simulink model "Target_Control_System"  (R2021b)
settings: Solver=FixedStepDiscrete  StartTime=0.0  StopTime=5  RelTol=1e-3
PreLoadFcn:
  | RTWConfigurationCB('preloadfcn', bdroot);
PostLoadFcn:
  | load('configuration/data_struct.mat');
  | load('configuration/fluxMaps_propMotor.mat');
  | load('configuration/parameterInit_PROP.mat');
  | load('configuration/parameterInit_PUMP.mat');
  | load('configuration/parameterInit_PITCH.mat');
  | load('configuration/parameterInit_TILT.mat');
  | %load('configuration/base_workspace_signal_definition.mat');
  | %load('resolvedatastores_to_baseworkspace_for_faster_simulation.mat');
model workspace (MAT data in the model file):
  SIMULATION_OPTIONS : Simulink.Parameter (value not decoded)
  TARGET_CODE_GEN : Simulink.Parameter (value not decoded)
  TCS_SAMPLE_FREQ_HZ : Simulink.Parameter (value not decoded)
symbols that are objects in the model workspace (value not decoded): TARGET_CODE_GEN, TCS_SAMPLE_FREQ_HZ
undefined symbols (not defined in the file): A_DQ_REF_LPF_INIT__PITCH, A_DQ_REF_LPF_INIT__PROP, A_DQ_REF_LPF_INIT__PUMP, A_DQ_REF_LPF_INIT__TILT, A_OBSERVER_CONFIDENCE_INIT__PITCH, A_OBSERVER_CONFIDENCE_INIT__PROP, A_OBSERVER_CONFIDENCE_INIT__PUMP, A_OBSERVER_CONFIDENCE_INIT__TILT, ACTUATOR_MAX_ANGLE_TRIP__PITCH, ACTUATOR_MIN_ANGLE_TRIP__PITCH, ACTUATOR_POS_SENSOR_INV_DIRECTION__PITCH, ACTUATOR_POS_SENSOR_INV_DIRECTION__TILT, ACTUATOR_POS_SENSOR_OFFSET__PITCH, ACTUATOR_POS_SENSOR_OFFSET__TILT, ADC_scaler1_baseaddr_TILT, ADC_SCALER_FLOAT_TO_FIXPOINT_EXPANSION, ANGLE_ELEC_FROM_SENSOR_OFFSET_INIT__PITCH, ANGLE_ELEC_FROM_SENSOR_OFFSET_INIT__PROP, ANGLE_ELEC_FROM_SENSOR_OFFSET_INIT__PUMP, ANGLE_ELEC_FROM_SENSOR_OFFSET_INIT__TILT, AUTO_CLEAR_FAULTS_ENABLED__PITCH, AUTO_CLEAR_FAULTS_ENABLED__PROP, AUTO_CLEAR_FAULTS_ENABLED__PUMP, AUTO_CLEAR_FAULTS_ENABLED__TILT, AUTO_CLEAR_FAULTS_WAIT_TICKS__PITCH, AUTO_CLEAR_FAULTS_WAIT_TICKS__PROP, AUTO_CLEAR_FAULTS_WAIT_TICKS__PUMP, AUTO_CLEAR_FAULTS_WAIT_TICKS__TILT, AUTO_I_ZERO_IDLE_TICKS__PITCH, AUTO_I_ZERO_IDLE_TICKS__PROP, AUTO_I_ZERO_IDLE_TICKS__PUMP, AUTO_I_ZERO_IDLE_TICKS__TILT, AUTO_I_ZERO_OFFSET_IDC_THRESHOLD__PITCH, AUTO_I_ZERO_OFFSET_IDC_THRESHOLD__PROP, AUTO_I_ZERO_OFFSET_IDC_THRESHOLD__PUMP, AUTO_I_ZERO_OFFSET_IDC_THRESHOLD__TILT, AUTO_I_ZERO_OFFSET_IPH_THRESHOLD__PITCH, AUTO_I_ZERO_OFFSET_IPH_THRESHOLD__PROP, AUTO_I_ZERO_OFFSET_IPH_THRESHOLD__PUMP, AUTO_I_ZERO_OFFSET_IPH_THRESHOLD__TILT, AUTO_SENSORLESS_SWITCHOVER_DISABLE_OMEGA, AUTO_SENSORLESS_SWITCHOVER_ENABLE_OMEGA, AUTO_SENSORLESS_SWITCHOVER_MIN_CONFIDENCE, AUXILIARY_PROTECTION_UNIT_BASEADDR__TILT, blanking_max_error_omega_INIT_PITCH, blanking_max_error_omega_INIT_TILT, blanking_max_error_position_INIT_PITCH, blanking_max_error_position_INIT_TILT, BRUTE_START_I_Q_REF_RAMP_SPEED__PITCH, BRUTE_START_I_Q_REF_RAMP_SPEED__PROP, BRUTE_START_I_Q_REF_RAMP_SPEED__PUMP, BRUTE_START_I_Q_REF_RAMP_SPEED__TILT, CONTROL_LOOP_DT_INIT__PITCH, CONTROL_LOOP_DT_INIT__PROP, CONTROL_LOOP_DT_INIT__PUMP, CONTROL_LOOP_DT_INIT__TILT, CORRECTION_FILTER_SCALE__PITCH, CORRECTION_FILTER_SCALE__PROP, CORRECTION_FILTER_SCALE__PUMP, CORRECTION_FILTER_SCALE__TILT ... (+458)
libraries: simulink x178, Reusables_Lib x24
(part 38 of 47)

== system Target_Control_System/Target_Control_System/MainLoop/tiltMotor_mainLoop/Decimation gate for 200 Hz Tilt/motorTaskMainDecimationAStep(&oTilt)/Forced current injection for broken input sensors/Enabled Subsystem/Rudimentary_forced_angle_position_control ==
  note: // (fErrorReduction_ assumed to be gte 0)
  note: // Limit maximum speed
  note: // Reduce top speed 33-fold
  Enable : EnablePort
  Abs : Abs
  Add : Sum  Inputs=+-
  Add1 : Sum  Inputs=+-
  Data Store Read10 : DataStoreRead  DataStoreName=oTilt  DataStoreElements=oTilt.oMot_.oState_.oPosSensor_.oPidDataPosCtrl_.oParameter_.fOutMax_  IndexOptions=Index vector (dialog)  Indices=1  OutputSizes=1
  Data Store Read11 : DataStoreRead  DataStoreName=oTilt  DataStoreElements=oTilt.oMot_.oState_.oPosSensor_.oPidDataPosCtrl_.oParameter_.fOutMin_  IndexOptions=Index vector (dialog)  Indices=1  OutputSizes=1
  Data Store Read6 : DataStoreRead  DataStoreName=oTilt  DataStoreElements=oTilt.oMot_.oState_.oRampDataPos_.fRampOut_  IndexOptions=Index vector (dialog)  Indices=1  OutputSizes=1
  Data Store Read7 : DataStoreRead  DataStoreName=oTilt  DataStoreElements=oTilt.oMot_.oState_.oPosSensor_.fActuatorAngleFromSensor_  IndexOptions=Index vector (dialog)  Indices=1  OutputSizes=1
  Data Store Read8 : DataStoreRead  DataStoreName=oTilt  DataStoreElements=oTilt.oMot_.oState_.oPosSensor_.oPidDataPosCtrl_.oParameter_.fErrorReduction_  IndexOptions=Index vector (dialog)  Indices=1  OutputSizes=1
  Data Store Read9 : DataStoreRead  DataStoreName=oTilt  DataStoreElements=oTilt.oMot_.oState_.oPosSensor_.oPidDataPosCtrl_.oParameter_.fKp_  IndexOptions=Index vector (dialog)  Indices=1  OutputSizes=1
  Data Store Write4 : DataStoreWrite  DataStoreName=oTilt  DataStoreElements=oTilt.oMot_.oState_.oRampDataOmegaERef_.fSetpoint_  IndexOptions=Index vector (dialog)  Indices=1  OutputSizes=1
  Divide : Product  Inputs=**
  Divide1 : Product  Inputs=**
  Gain : Gain  Gain=0.03
  Gain1 : Gain  Gain=0.03
  Max : MinMax  Function=max  Inputs=2
  Min : MinMax  Inputs=2
  Saturation : Saturate  UpperLimit=inf  LowerLimit=0
  Sign : Signum
  wires:
  Data Store Read10/1 -> Gain/1
  Gain/1 -> Min/2
  Data Store Read9/1 -> Divide1/2
  Divide1/1 -> Min/1  "fOmegaRef"
  Sign/1 -> Divide/1
  Data Store Read11/1 -> Gain1/1
  Saturation/1 -> Divide/2
  Min/1 -> Max/1
  Gain1/1 -> Max/2
  Data Store Read7/1 -> Add/2
  Add1/1 -> Saturation/1  "fTemp"
  Data Store Read8/1 -> Add1/2
  Add/1 -> Abs/1, Sign/1  "fPositionError"
  Divide/1 -> Divide1/1  "fPositionError"
  Data Store Read6/1 -> Add/1
  Abs/1 -> Add1/1
  Max/1 -> Data Store Write4/1

== system Target_Control_System/Target_Control_System/MainLoop/tiltMotor_mainLoop/Decimation gate for 200 Hz Tilt/motorTaskMainDecimationAStep(&oTilt)/Idle controller/Not forced angle/piControllerStep_Idle_Controller(&oTilt) ==
  fActual : Inport
  fTarget : Inport  Port=2
  fKp : Inport  Port=3
  fKi : Inport  Port=4
  fScale : Inport  Port=5
  fLoopDt : Inport  Port=6
  fIntMax : Inport  Port=7
  fOutMax : Inport  Port=8
  fIntMin : Inport  Port=9
  fOutMin : Inport  Port=10
  fState : Inport  Port=11
  Add : Sum  Inputs=|++
  Mux : Mux  Inputs=3
  Mux1 : Mux  Inputs=3
  Product : Product
  Saturation Dynamic : simulink/Discontinuities/Saturation Dynamic  OutMin=[]  OutMax=[]  OutDataTypeStr=Inherit: Same as second input  OutDataType=fixdt(1, 16)  OutScaling=2^-10  DoSatur=off
  Saturation Dynamic1 : simulink/Discontinuities/Saturation Dynamic  OutMin=[]  OutMax=[]  OutDataTypeStr=Inherit: Same as second input  OutDataType=fixdt(1, 16)  OutScaling=2^-10  DoSatur=off
  Scope3 : Scope  NumInputPorts=6
  Sum1 : Sum  Inputs=++|
  Sum22 : Sum  Inputs=-+|
  Unit Delay2 : UnitDelay  SampleTime=-1  HasFrameUpgradeWarning=on
  fError * fKi_ * fScale : Fcn  Expr=u(1)*u(2)*u(3)
  fError * fKp_ * fScale1 : Fcn  Expr=u(1)*u(2)*u(3)
  fOutput : Outport
  *fpState : Outport  Port=2
  wires:
  fLoopDt/1 -> Product/2
  fOutMax/1 -> Saturation Dynamic1/1
  fOutMin/1 -> Saturation Dynamic1/3
  fIntMin/1 -> Saturation Dynamic/3
  fIntMax/1 -> Saturation Dynamic/1
  Unit Delay2/1 -> Scope3/5, *fpState/1, Sum1/2
  Add/1 -> Saturation Dynamic/2
  fState/1 -> Add/2
  Product/1 -> Add/1
  Mux1/1 -> fError * fKp_ * fScale1/1
  fKi/1 -> Mux/2
  fScale/1 -> Mux/1, Mux1/3
  fKp/1 -> Mux1/2
  Mux/1 -> fError * fKi_ * fScale/1
  Saturation Dynamic1/1 -> fOutput/1, Scope3/6
  Sum1/1 -> Saturation Dynamic1/2  "fError"
  fError * fKp_ * fScale1/1 -> Sum1/1, Scope3/4
  Saturation Dynamic/1 -> Unit Delay2/1  "*fpState"
  fActual/1 -> Sum22/1, Scope3/2
  fTarget/1 -> Sum22/2, Scope3/1
  fError * fKi_ * fScale/1 -> Product/1
  Sum22/1 -> Scope3/3, Mux/3, Mux1/1  "fError"

== system Target_Control_System/Target_Control_System/MainLoop/tiltMotor_mainLoop/Decimation gate for 200 Hz Tilt/motorTaskMainDecimationAStep(&oTilt)/Position control checks/Position control mode/Check AD2S1210 ==
  function : TriggerPort  TriggerType=function-call  VariantControl=Variant
  Data Store Read : DataStoreRead  DataStoreName=oTilt  DataStoreElements=oTilt.oMot_.oState_.oPosSensor_.eInputPositionSensorType_  IndexOptions=Index vector (dialog)  Indices=1  OutputSizes=1
  Enabled Subsystem : Subsystem  TreatAsAtomicUnit=on
  Enumerated Constant : simulink/Sources/Enumerated Constant  OutDataTypeStr=Enum: EPositionSensor_t  Value=EPositionSensor_t.eResolver  SampleTime=-1
  Equal : RelationalOperator  Operator===  OutDataTypeStr=boolean  RndMeth=Simplest
  wires:
  Equal/1 -> Enabled Subsystem/Enable
  Data Store Read/1 -> Equal/1
  Enumerated Constant/1 -> Equal/2

== system Target_Control_System/Target_Control_System/MainLoop/tiltMotor_mainLoop/Decimation gate for 200 Hz Tilt/motorTaskMainDecimationAStep(&oTilt)/Position control checks/Position control mode/Check fighting controllers ==
  note: Check fighting controllers
      | (For dual inverter independent position control)
      | MvdG: Possibly remove again, because it is not actually in use? QAZ
  note: (ab)use the threshold setting as on-off switch too.
  function : TriggerPort  TriggerType=function-call  VariantControl=Variant
  Constant : Constant  Value=0  OutDataTypeStr=int32  SampleTime=-1
  Data Store Read : DataStoreRead  DataStoreName=oTilt  DataStoreElements=oTilt.oMot_.oState_.oPosSensor_.fFightingCurrentMagnitude_  IndexOptions=Index vector (dialog)  Indices=1  OutputSizes=1
  Enabled Subsystem : Subsystem  TreatAsAtomicUnit=on
  GreaterThan : RelationalOperator  Operator=>  OutDataTypeStr=boolean  RndMeth=Simplest
  wires:
  Constant/1 -> GreaterThan/2
  GreaterThan/1 -> Enabled Subsystem/Enable
  Data Store Read/1 -> GreaterThan/1

== system Target_Control_System/Target_Control_System/MainLoop/tiltMotor_mainLoop/Decimation gate for 200 Hz Tilt/motorTaskMainDecimationAStep(&oTilt)/Position control checks/Position control mode/Check for position halted ==
  function : TriggerPort  TriggerType=function-call  VariantControl=Variant
  Chart1 : Stateflow chart  TreatAsAtomicUnit=on

== system Target_Control_System/Target_Control_System/MainLoop/tiltMotor_mainLoop/Decimation gate for 200 Hz Tilt/motorTaskMainDecimationAStep(&oTilt)/Position control checks/Position control mode/checkSensorLimits(&oTilt) ==
  note: In the emergency 'ePassiveHolding' mode, iPosControlEnabled_ is false, so this will not trip
  function : TriggerPort  TriggerType=function-call  VariantControl=Variant
  Check broken sensor : Subsystem  TreatAsAtomicUnit=on
  Check delta input-output : Subsystem  TreatAsAtomicUnit=on
  Check for stuck sensor : Subsystem  TreatAsAtomicUnit=on
  Check limits : Subsystem  TreatAsAtomicUnit=on
  Function-Call Generator : simulink/Ports & Subsystems/Function-Call Generator  sample_time=-1  numberOfIterations=1  DisallowWideOutput=off
  Function-Call Split{1..3,10} (4 alike) : FunctionCallSplit  NumOutputPorts=2
  Read sensor flags : Subsystem  TreatAsAtomicUnit=on
  wires:
  Function-Call Split2/2 -> Function-Call Split3/1
  Function-Call Split10/1 -> Read sensor flags/Trigger
  Function-Call Split1/1 -> Check limits/Trigger
  Function-Call Split3/2 -> Check for stuck sensor/Trigger
  Function-Call Split1/2 -> Function-Call Split2/1
  Function-Call Split2/1 -> Check broken sensor/Trigger
  Function-Call Generator/1 -> Function-Call Split10/1
  Function-Call Split3/1 -> Check delta input-output/Trigger
  Function-Call Split10/2 -> Function-Call Split1/1

== system Target_Control_System/Target_Control_System/MainLoop/tiltMotor_mainLoop/Decimation gate for 5000 Hz Tilt/motorTaskProcessExternalSetpoints(&oTilt)/set_target/Id_target/Subsystem ==
  Input : Inport
  Enable : EnablePort
  Data Store Read1 : DataStoreRead  DataStoreName=oTilt  DataStoreElements=oTilt.oMot_.oParam_.fISetpointMax_  IndexOptions=Index vector (dialog)  Indices=1  OutputSizes=1
  Data Store Read74 : DataStoreRead  DataStoreName=oTilt  DataStoreElements=oTilt.oMot_.oParam_.fISetpointMax_  IndexOptions=Index vector (dialog)  Indices=1  OutputSizes=1
  Data Store Write1 : DataStoreWrite  DataStoreName=oTilt  DataStoreElements=oTilt.oMot_.oState_.fIdExternalSetpoint_  IndexOptions=Index vector (dialog)  Indices=1  OutputSizes=1
  Gain2 : Gain  Gain=-1
  Saturation Dynamic : simulink/Discontinuities/Saturation Dynamic  OutMin=[]  OutMax=[]  OutDataTypeStr=Inherit: Same as second input  OutDataType=fixdt(1, 16)  OutScaling=2^-10  DoSatur=off
  wires:
  Data Store Read1/1 -> Gain2/1
  Data Store Read74/1 -> Saturation Dynamic/1
  Gain2/1 -> Saturation Dynamic/3
  Input/1 -> Saturation Dynamic/2
  Saturation Dynamic/1 -> Data Store Write1/1

== system Target_Control_System/Target_Control_System/MainLoop/tiltMotor_mainLoop/Decimation gate for 5000 Hz Tilt/motorTaskProcessExternalSetpoints(&oTilt)/set_target/Iq_target/Subsystem ==
  Enable : EnablePort
  Data Store Read1 : DataStoreRead  DataStoreName=oTilt  DataStoreElements=oTilt.oMot_.oParam_.fIqSetpointMax_  IndexOptions=Index vector (dialog)  Indices=1  OutputSizes=1
  Data Store Read68 : DataStoreRead  DataStoreName=oTilt  DataStoreElements=oTilt.oMot_.oIn_.fIqSetpoint_  IndexOptions=Index vector (dialog)  Indices=1  OutputSizes=1
  Data Store Read74 : DataStoreRead  DataStoreName=oTilt  DataStoreElements=oTilt.oMot_.oParam_.fIqSetpointMax_  IndexOptions=Index vector (dialog)  Indices=1  OutputSizes=1
  Data Store Read81 : DataStoreRead  DataStoreName=oTilt  DataStoreElements=oTilt.oMot_.oParam_.fDynILimIntegratorLeakageFactor_  IndexOptions=Index vector (dialog)  Indices=1  OutputSizes=1
  Data Store Write19 : DataStoreWrite  DataStoreName=oTilt  DataStoreElements=oTilt.oMot_.oState_.fIqRefBeforeRamp_  IndexOptions=Index vector (dialog)  Indices=1  OutputSizes=1
  Dynamic Current Limiting Tilt : Subsystem  TreatAsAtomicUnit=on
  Gain2 : Gain  Gain=-1
  Saturation Dynamic : simulink/Discontinuities/Saturation Dynamic  OutMin=[]  OutMax=[]  OutDataTypeStr=Inherit: Same as second input  OutDataType=fixdt(1, 16)  OutScaling=2^-10  DoSatur=off
  Switch4 : Switch  Criteria=u2 > Threshold
  wires:
  Dynamic Current Limiting Tilt/1(fIqRefBeforeRamp_) -> Switch4/1
  Switch4/1 -> Data Store Write19/1
  Data Store Read81/1 -> Dynamic Current Limiting Tilt/Enable, Switch4/2
  Gain2/1 -> Saturation Dynamic/3
  Data Store Read74/1 -> Saturation Dynamic/1
  Data Store Read68/1 -> Saturation Dynamic/2
  Data Store Read1/1 -> Gain2/1
  Saturation Dynamic/1 -> Switch4/3

== system Target_Control_System/Target_Control_System/MainLoop/tiltMotor_mainLoop/Decimation gate for 5000 Hz Tilt/motorTaskProcessExternalSetpoints(&oTilt)/set_target/position_target/Subsystem ==
  Enable : EnablePort
  Data Store Read2 : DataStoreRead  DataStoreName=oTilt  DataStoreElements=oTilt.oMot_.oIn_.fPosSetpoint_  IndexOptions=Index vector (dialog)  Indices=1  OutputSizes=1
  Data Store Read85 : DataStoreRead  DataStoreName=oTilt  DataStoreElements=oTilt.oMot_.oState_.uiDriveState_  IndexOptions=Index vector (dialog)  Indices=1  OutputSizes=1
  Data Store Write1 : DataStoreWrite  DataStoreName=oTilt  DataStoreElements=oTilt.oMot_.oState_.oRampDataPos_.fSetpoint_  IndexOptions=Index vector (dialog)  Indices=1  OutputSizes=1
  Equal13 : RelationalOperator  Operator=~=  OutDataTypeStr=boolean  RndMeth=Simplest
  Position Limiting Tilt : Subsystem  TreatAsAtomicUnit=on
  const17 : Constant  Value=228  OutDataTypeStr=uint32  SampleTime=-1
  wires:
  Equal13/1 -> Position Limiting Tilt/Enable
  const17/1 -> Equal13/1
  Data Store Read85/1 -> Equal13/2
  Data Store Read2/1 -> Data Store Write1/1, Position Limiting Tilt/1(oRampDataPos_.fSetpoint_)

== system Target_Control_System/Target_Control_System/MainLoop/tiltMotor_mainLoop/Decimation gate for 5000 Hz Tilt/motorTaskProcessExternalSetpoints(&oTilt)/set_target/speed_target/Subsystem ==
  Enable : EnablePort
  Data Store Read1 : DataStoreRead  DataStoreName=oTilt  DataStoreElements=oTilt.oMot_.oParam_.fPolePairs_  IndexOptions=Index vector (dialog)  Indices=1  OutputSizes=1
  Data Store Read2 : DataStoreRead  DataStoreName=oTilt  DataStoreElements=oTilt.oMot_.oIn_.fRpmSetpoint_  IndexOptions=Index vector (dialog)  Indices=1  OutputSizes=1
  Data Store Read3 : DataStoreRead  DataStoreName=oTilt  DataStoreElements=oTilt.oMot_.oParam_.fOmegaESetpointMax_  IndexOptions=Index vector (dialog)  Indices=1  OutputSizes=1
  Data Store Read74 : DataStoreRead  DataStoreName=oTilt  DataStoreElements=oTilt.oMot_.oParam_.fOmegaESetpointMax_  IndexOptions=Index vector (dialog)  Indices=1  OutputSizes=1
  Data Store Write1 : DataStoreWrite  DataStoreName=oTilt  DataStoreElements=oTilt.oMot_.oState_.oRampDataOmegaERef_.fSetpoint_  IndexOptions=Index vector (dialog)  Indices=1  OutputSizes=1
  Gain : Gain  Gain=-1
  Product : Product  Inputs=3
  Saturation Dynamic : simulink/Discontinuities/Saturation Dynamic  OutMin=[]  OutMax=[]  OutDataTypeStr=Inherit: Same as second input  OutDataType=fixdt(1, 16)  OutScaling=2^-10  DoSatur=off
  const1 : Constant  Value=0.10471975512  OutDataTypeStr=single  SampleTime=-1
  wires:
  Saturation Dynamic/1 -> Data Store Write1/1
  Product/1 -> Saturation Dynamic/2
  Data Store Read3/1 -> Gain/1
  Gain/1 -> Saturation Dynamic/3
  Data Store Read74/1 -> Saturation Dynamic/1
  const1/1 -> Product/2
  Data Store Read1/1 -> Product/3
  Data Store Read2/1 -> Product/1

== system Target_Control_System/Target_Control_System/MainLoop/tiltMotor_mainLoop/mainTask_tilt/motorTaskMainFastStep(&oTilt)/Automatic switching to sensorless - Tilt/Automatic switching to sensorless/Switch to sensored  ==
  note: // Presently enabled, do we need to disable?
  fObserverConfidence : Inport
  Action Port : ActionPort
  Abs2 : Abs
  Data Store Read1 : DataStoreRead  DataStoreName=oTilt  DataStoreElements=oTilt.oMot_.oIn_.fOmegaEObserverRaw2_  IndexOptions=Index vector (dialog)  Indices=1  OutputSizes=1
  Data Store Read2 : DataStoreRead  DataStoreName=oTilt  DataStoreElements=oTilt.oMot_.oParam_.fAutoSensorlessSwitchoverDisableOmega_  IndexOptions=Index vector (dialog)  Indices=1  OutputSizes=1
  Data Store Read3 : DataStoreRead  DataStoreName=oTilt  DataStoreElements=oTilt.oMot_.oParam_.fAutoSensorlessSwitchoverMinConfidence_  IndexOptions=Index vector (dialog)  Indices=1  OutputSizes=1
  Less Than2 : RelationalOperator  Operator=<  OutDataTypeStr=boolean  RndMeth=Simplest
  Less Than3 : RelationalOperator  Operator=<  OutDataTypeStr=boolean  RndMeth=Simplest
  OR1 : Logic  Operator=OR  AllPortsSameDT=off  OutDataTypeStr=boolean
  Switch to sensored : Subsystem  TreatAsAtomicUnit=on
  wires:
  Data Store Read2/1 -> Less Than2/2
  Data Store Read3/1 -> Less Than3/2
  OR1/1 -> Switch to sensored/Enable
  Less Than3/1 -> OR1/2
  fObserverConfidence/1 -> Less Than3/1
  Abs2/1 -> Less Than2/1
  Less Than2/1 -> OR1/1
  Data Store Read1/1 -> Abs2/1

== system Target_Control_System/Target_Control_System/MainLoop/tiltMotor_mainLoop/mainTask_tilt/motorTaskMainFastStep(&oTilt)/Automatic switching to sensorless - Tilt/Automatic switching to sensorless/Switch to sensorless? ==
  fObserverConfidence : Inport
  Action Port : ActionPort
  Abs2 : Abs
  Data Store Read1 : DataStoreRead  DataStoreName=oTilt  DataStoreElements=oTilt.oMot_.oIn_.fOmegaEObserverRaw2_  IndexOptions=Index vector (dialog)  Indices=1  OutputSizes=1
  Data Store Read2 : DataStoreRead  DataStoreName=oTilt  DataStoreElements=oTilt.oMot_.oParam_.fAutoSensorlessSwitchoverEnableOmega_  IndexOptions=Index vector (dialog)  Indices=1  OutputSizes=1
  Data Store Read3 : DataStoreRead  DataStoreName=oTilt  DataStoreElements=oTilt.oMot_.oParam_.fAutoSensorlessSwitchoverMinConfidence_  IndexOptions=Index vector (dialog)  Indices=1  OutputSizes=1
  Less Than2 : RelationalOperator  Operator=>  OutDataTypeStr=boolean  RndMeth=Simplest
  Less Than3 : RelationalOperator  Operator=>  OutDataTypeStr=boolean  RndMeth=Simplest
  OR1 : Logic  AllPortsSameDT=off  OutDataTypeStr=boolean
  Switch to sensorless : Subsystem  TreatAsAtomicUnit=on
  wires:
  OR1/1 -> Switch to sensorless/Enable
  Data Store Read3/1 -> Less Than3/2
  Less Than2/1 -> OR1/1
  Data Store Read2/1 -> Less Than2/2
  Data Store Read1/1 -> Abs2/1
  Abs2/1 -> Less Than2/1
  fObserverConfidence/1 -> Less Than3/1
  Less Than3/1 -> OR1/2

== system Target_Control_System/Target_Control_System/MainLoop/tiltMotor_mainLoop/mainTask_tilt/motorTaskMainFastStep(&oTilt)/Control Loops - Tilt/Position Controller Tilt/Connect PosController to CurrentController ==
  fPMultiplier : Inport
  fIMultiplier : Inport  Port=2
  DMultiplier : Inport  Port=3
  fITerm : Inport  Port=4
  fDTerm : Inport  Port=5
  fPTerm : Inport  Port=6
  Add : Sum  Inputs=+++
  Divide : Product  Inputs=**
  Divide1 : Product  Inputs=**
  Divide2 : Product  Inputs=**
  fIqRefFromSpeedController : Outport
  wires:
  Add/1 -> fIqRefFromSpeedController/1
  Divide2/1 -> Add/3
  Divide/1 -> Add/1
  Divide1/1 -> Add/2
  fDTerm/1 -> Divide2/1
  DMultiplier/1 -> Divide2/2
  fITerm/1 -> Divide1/1
  fIMultiplier/1 -> Divide1/2
  fPMultiplier/1 -> Divide/2
  fPTerm/1 -> Divide/1

== system Target_Control_System/Target_Control_System/MainLoop/tiltMotor_mainLoop/mainTask_tilt/motorTaskMainFastStep(&oTilt)/Control Loops - Tilt/Position Controller Tilt/pid2ControllerStep(oPidDataPosCtrl)_pitch ==
  fTarget : Inport
  fActual : Inport  Port=2
  fErrorReduction : Inport  Port=3
  fLargeErrorThresholdPositive : Inport  Port=4
  fLargeErrorThresholdNegative : Inport  Port=5
  fBlankingMaxError : Inport  Port=6
  fKi : Inport  Port=7
  ipInhibitTarget : Inport  Port=8
  fLoopDt : Inport  Port=9
  fIntMax : Inport  Port=10
  fIntMin : Inport  Port=11
  fIntegratorLeakFactor : Inport  Port=12
  fKd : Inport  Port=13
  fActualDt : Inport  Port=14
  fDMax : Inport  Port=15
  fDMin : Inport  Port=16
  fKp : Inport  Port=17
  fOutMax : Inport  Port=18
  fOutMin : Inport  Port=19
  fpState : Inport  Port=20
  Abs : Abs
  Abs1 : Abs
  Add : Sum  Inputs=|++
  Add1 : Sum
  Constant : Constant  Value=0  OutDataTypeStr=single  SampleTime=-1
  Constant3 : Constant  Value=0  OutDataTypeStr=single  SampleTime=-1
  Constant4 : Constant  Value=0  OutDataTypeStr=single  SampleTime=-1
  Constant5 : Constant  OutDataTypeStr=single  SampleTime=-1
  Constant6 : Constant  OutDataTypeStr=int32  SampleTime=-1
  Constant7 : Constant  Value=-1  OutDataTypeStr=int32  SampleTime=-1
  Constant8 : Constant  Value=0  OutDataTypeStr=int32  SampleTime=-1
  Divide : Product  Inputs=**
  Divide1 : Product  Inputs=**
  GreaterThan2 : RelationalOperator  OutDataTypeStr=boolean  RndMeth=Simplest
  GreaterThan3 : RelationalOperator  Operator=>  OutDataTypeStr=boolean  RndMeth=Simplest
  GreaterThan4 : RelationalOperator  Operator=>  OutDataTypeStr=boolean  RndMeth=Simplest
  GreaterThan5 : RelationalOperator  Operator=<  OutDataTypeStr=boolean  RndMeth=Simplest
  GreaterThan6 : RelationalOperator  Operator=<  OutDataTypeStr=boolean  RndMeth=Simplest
  GreaterThan7 : RelationalOperator  Operator=>  OutDataTypeStr=boolean  RndMeth=Simplest
  GreaterThan8 : RelationalOperator  Operator=<  OutDataTypeStr=boolean  RndMeth=Simplest
  OR1 : Logic  AllPortsSameDT=off  OutDataTypeStr=boolean
  OR2 : Logic  AllPortsSameDT=off  OutDataTypeStr=boolean
  OR3 : Logic  Operator=OR  AllPortsSameDT=off  OutDataTypeStr=boolean
  Product{,1..4} (5 alike) : Product
  Saturation : Saturate  UpperLimit=inf  LowerLimit=0
  Saturation Dynamic : simulink/Discontinuities/Saturation Dynamic  OutMin=[]  OutMax=[]  OutDataTypeStr=Inherit: Same as second input  OutDataType=fixdt(1, 16)  OutScaling=2^-10  DoSatur=off
  Saturation Dynamic1 : simulink/Discontinuities/Saturation Dynamic  OutMin=[]  OutMax=[]  OutDataTypeStr=Inherit: Same as second input  OutDataType=fixdt(1, 16)  OutScaling=2^-10  DoSatur=off
  Saturation Dynamic2 : simulink/Discontinuities/Saturation Dynamic  OutMin=[]  OutMax=[]  OutDataTypeStr=Inherit: Same as second input  OutDataType=fixdt(1, 16)  OutScaling=2^-10  DoSatur=off
  Scope : Scope  NumInputPorts=4
  Sign : Signum
  Sum : Sum  Inputs=|++
  Sum2 : Sum  Inputs=-+|
  Sum22 : Sum  Inputs=-+|
  Sum4 : Sum  Inputs=+-|
  Switch{1..4} (4 alike) : Switch  Criteria=u2 > Threshold
  Unit Delay2 : UnitDelay  SampleTime=-1  HasFrameUpgradeWarning=on
  iLargeErrorPresent : Outport
  fITerm : Outport  Port=2
  fDTerm : Outport  Port=3
  fPTerm : Outport  Port=4
  fOutput : Outport  Port=5
  *fpState : Outport  Port=6
  wires:
  Switch3/1 -> iLargeErrorPresent/1
  Constant6/1 -> Switch4/1
  GreaterThan8/1 -> Switch3/2
  GreaterThan7/1 -> Switch4/2
  Switch4/1 -> Switch3/3
  Constant8/1 -> Switch4/3
  Constant7/1 -> Switch3/1
  Sum/1 -> Saturation Dynamic1/2, Scope/2
  Add1/1 -> Sum/2
  Product4/1 -> fPTerm/1, Sum/1
  fKp/1 -> Product4/1
  Saturation Dynamic2/1 -> fDTerm/1, Add1/1  "fDTerm"
  fDMax/1 -> Saturation Dynamic2/1
  fDMin/1 -> Saturation Dynamic2/3
  Product3/1 -> Saturation Dynamic2/2  "fDTerm"
  fActualDt/1 -> Product3/2
  fKd/1 -> Product3/1
  Unit Delay2/1 -> Product2/1  "*fpState"
  Product2/1 -> fITerm/1, *fpState/1, Add1/2  "*fpState"
  Sum4/1 -> Product2/2
  Constant5/1 -> Sum4/1
  Product1/1 -> Sum4/2
  fIntegratorLeakFactor/1 -> Product1/2
  Saturation Dynamic/1 -> Unit Delay2/1
  Add/1 -> Saturation Dynamic/2  "fpState"
  Switch2/1 -> Product/1  "fErrorForIntegrator"
  Constant4/1 -> Switch2/1
  OR3/1 -> Switch2/2
  OR2/1 -> OR3/2
  OR1/1 -> OR3/1
  GreaterThan6/1 -> OR2/2
  GreaterThan5/1 -> OR2/1
  GreaterThan3/1 -> OR1/2
  GreaterThan4/1 -> OR1/1
  Divide1/1 -> GreaterThan4/1, Switch2/3, GreaterThan5/1  "fErrorForIntegrator"
  Constant3/1 -> GreaterThan3/2, GreaterThan4/2, GreaterThan5/2, GreaterThan6/2
  ipInhibitTarget/1 -> GreaterThan6/1, GreaterThan3/1
  fKi/1 -> Divide1/2
  Switch1/1 -> Divide1/1  "fErrorForIntegrator"
  Constant/1 -> Switch1/3
  GreaterThan2/1 -> Switch1/2
  fBlankingMaxError/1 -> GreaterThan2/2
  Abs1/1 -> GreaterThan2/1
  fLargeErrorThresholdNegative/1 -> GreaterThan8/2
  fLargeErrorThresholdPositive/1 -> GreaterThan7/2
  Divide/1 -> Product4/2, GreaterThan8/1, Abs1/1, Switch1/1, GreaterThan7/1  "fError"
  Sign/1 -> Divide/2
  Saturation/1 -> Divide/1
  Sum2/1 -> Saturation/1  "fTemp"
  fErrorReduction/1 -> Sum2/1
  Abs/1 -> Sum2/2
  fActual/1 -> Sum22/1
  fOutMax/1 -> Saturation Dynamic1/1, Scope/3
  fpState/1 -> Add/2
  Saturation Dynamic1/1 -> fOutput/1, Scope/1
  fTarget/1 -> Sum22/2
  Product/1 -> Add/1
  Sum22/1 -> Abs/1, Sign/1  "fError"
  fOutMin/1 -> Saturation Dynamic1/3, Scope/4
  fIntMax/1 -> Saturation Dynamic/1
  fLoopDt/1 -> Product/2, Product1/1
  fIntMin/1 -> Saturation Dynamic/3

== system Target_Control_System/Target_Control_System/MainLoop/tiltMotor_mainLoop/mainTask_tilt/motorTaskMainFastStep(&oTilt)/Control Loops - Tilt/Speed Controller Tilt/PID2controller_sensoredDrives ==
  oRampDataOmegaERef_.fRampOut : Inport
  Enable : EnablePort
  Constant1 : Constant  OutDataTypeStr=single  SampleTime=-1
  Data Store Read10 : DataStoreRead  DataStoreName=oTilt  DataStoreElements=oTilt.oMot_.oParam_.oPid2DataRpmCtrl_.oParameter_.fLargeErrorThresholdNegative_  IndexOptions=Index vector (dialog)  Indices=1  OutputSizes=1
  Data Store Read12 : DataStoreRead  DataStoreName=oTilt  DataStoreElements=oTilt.oMot_.oParam_.oPid2DataRpmCtrl_.oParameter_.fBlankingMaxError_  IndexOptions=Index vector (dialog)  Indices=1  OutputSizes=1
  Data Store Read14 : DataStoreRead  DataStoreName=oTilt  DataStoreElements=oTilt.oMot_.oParam_.oPid2DataRpmCtrl_.oParameter_.fKi_  IndexOptions=Index vector (dialog)  Indices=1  OutputSizes=1
  Data Store Read15 : DataStoreRead  DataStoreName=oTilt  DataStoreElements=oTilt.oMot_.oParam_.oPid2DataRpmCtrl_.oParameter_.fLoopDt_  IndexOptions=Index vector (dialog)  Indices=1  OutputSizes=1
  Data Store Read16 : DataStoreRead  DataStoreName=oTilt  DataStoreElements=oTilt.oMot_.oParam_.oPid2DataRpmCtrl_.oParameter_.fIntMax_  IndexOptions=Index vector (dialog)  Indices=1  OutputSizes=1
  Data Store Read17 : DataStoreRead  DataStoreName=oTilt  DataStoreElements=oTilt.oMot_.oParam_.oPid2DataRpmCtrl_.oParameter_.fIntMin_  IndexOptions=Index vector (dialog)  Indices=1  OutputSizes=1
  Data Store Read18 : DataStoreRead  DataStoreName=oTilt  DataStoreElements=oTilt.oMot_.oParam_.oPid2DataRpmCtrl_.oParameter_.ipInhibitTarget_  IndexOptions=Index vector (dialog)  Indices=1  OutputSizes=1
  Data Store Read19 : DataStoreRead  DataStoreName=oTilt  DataStoreElements=oTilt.oMot_.oParam_.oPid2DataRpmCtrl_.oParameter_.fIntegratorLeakFactor_  IndexOptions=Index vector (dialog)  Indices=1  OutputSizes=1
  Data Store Read20 : DataStoreRead  DataStoreName=oTilt  DataStoreElements=oTilt.oMot_.oParam_.oPid2DataRpmCtrl_.oParameter_.fKd_  IndexOptions=Index vector (dialog)  Indices=1  OutputSizes=1
  Data Store Read21 : DataStoreRead  DataStoreName=oTilt  DataStoreElements=oTilt.oMot_.oParam_.oPid2DataRpmCtrl_.oParameter_.fDMax_  IndexOptions=Index vector (dialog)  Indices=1  OutputSizes=1
  Data Store Read22 : DataStoreRead  DataStoreName=oTilt  DataStoreElements=oTilt.oMot_.oParam_.oPid2DataRpmCtrl_.oParameter_.fDMin_  IndexOptions=Index vector (dialog)  Indices=1  OutputSizes=1
  Data Store Read23 : DataStoreRead  DataStoreName=oTilt  DataStoreElements=oTilt.oMot_.oParam_.oPid2DataRpmCtrl_.oParameter_.fKp_  IndexOptions=Index vector (dialog)  Indices=1  OutputSizes=1
  Data Store Read24 : DataStoreRead  DataStoreName=oTilt  DataStoreElements=oTilt.oMot_.oParam_.oPid2DataRpmCtrl_.oParameter_.fOutMin_  IndexOptions=Index vector (dialog)  Indices=1  OutputSizes=1
  Data Store Read3 : DataStoreRead  DataStoreName=oTilt  DataStoreElements=oTilt.oMot_.oParam_.oPid2DataRpmCtrl_.oParameter_.fOutMax_  IndexOptions=Index vector (dialog)  Indices=1  OutputSizes=1
  Data Store Read4 : DataStoreRead  DataStoreName=oTilt  DataStoreElements=oTilt.oMot_.oParam_.oPid2DataRpmCtrl_.fState_  IndexOptions=Index vector (dialog)  Indices=1  OutputSizes=1
  Data Store Read7 : DataStoreRead  DataStoreName=oTilt  DataStoreElements=oTilt.oMot_.oState_.oPosSensor_.fOmegaEFromSensor_  IndexOptions=Index vector (dialog)  Indices=1  OutputSizes=1
  Data Store Read8 : DataStoreRead  DataStoreName=oTilt  DataStoreElements=oTilt.oMot_.oParam_.oPid2DataRpmCtrl_.oParameter_.fErrorReduction_  IndexOptions=Index vector (dialog)  Indices=1  OutputSizes=1
  Data Store Read9 : DataStoreRead  DataStoreName=oTilt  DataStoreElements=oTilt.oMot_.oParam_.oPid2DataRpmCtrl_.oParameter_.fLargeErrorThresholdPositive_  IndexOptions=Index vector (dialog)  Indices=1  OutputSizes=1
  Data Store Write : DataStoreWrite  DataStoreName=oTilt  DataStoreElements=oTilt.oMot_.oParam_.oPid2DataRpmCtrl_.oParameter_.iLargeErrorPresent_  IndexOptions=Index vector (dialog)  Indices=1  OutputSizes=1
  Data Store Write1 : DataStoreWrite  DataStoreName=oTilt  DataStoreElements=oTilt.oMot_.oParam_.oPid2DataRpmCtrl_.oParameter_.fITerm_  IndexOptions=Index vector (dialog)  Indices=1  OutputSizes=1
  Data Store Write2 : DataStoreWrite  DataStoreName=oTilt  DataStoreElements=oTilt.oMot_.oParam_.oPid2DataRpmCtrl_.oParameter_.fDTerm_  IndexOptions=Index vector (dialog)  Indices=1  OutputSizes=1
  Data Store Write3 : DataStoreWrite  DataStoreName=oTilt  DataStoreElements=oTilt.oMot_.oParam_.oPid2DataRpmCtrl_.oParameter_.fPTerm_  IndexOptions=Index vector (dialog)  Indices=1  OutputSizes=1
  Data Store Write4 : DataStoreWrite  DataStoreName=oTilt  DataStoreElements=oTilt.oMot_.oState_.fIqRefFromSpeedController_  IndexOptions=Index vector (dialog)  Indices=1  OutputSizes=1
  Data Store Write5 : DataStoreWrite  DataStoreName=oTilt  DataStoreElements=oTilt.oMot_.oParam_.oPid2DataRpmCtrl_.fState_  IndexOptions=Index vector (dialog)  Indices=1  OutputSizes=1
  pid2ControllerStep(oPidDataRpmCtrll_tilt : Subsystem  TreatAsAtomicUnit=on
  fIqRefFromSpeedController : Outport
  wires:
  oRampDataOmegaERef_.fRampOut/1 -> pid2ControllerStep(oPidDataRpmCtrll_tilt/2(fTarget)
  Data Store Read17/1 -> pid2ControllerStep(oPidDataRpmCtrll_tilt/11(fIntMin)
  Data Store Read20/1 -> pid2ControllerStep(oPidDataRpmCtrll_tilt/13(fKd)
  Data Store Read10/1 -> pid2ControllerStep(oPidDataRpmCtrll_tilt/5(fLargeErrorThresholdNegative)
  Data Store Read22/1 -> pid2ControllerStep(oPidDataRpmCtrll_tilt/16(fDMin)
  pid2ControllerStep(oPidDataRpmCtrll_tilt/5(fOutput) -> Data Store Write4/1, fIqRefFromSpeedController/1
  Data Store Read18/1 -> pid2ControllerStep(oPidDataRpmCtrll_tilt/8(ipInhibitTarget)
  pid2ControllerStep(oPidDataRpmCtrll_tilt/4(fPTerm) -> Data Store Write3/1
  Data Store Read15/1 -> pid2ControllerStep(oPidDataRpmCtrll_tilt/9(fLoopDt)
  Data Store Read14/1 -> pid2ControllerStep(oPidDataRpmCtrll_tilt/7(fKi)
  Data Store Read8/1 -> pid2ControllerStep(oPidDataRpmCtrll_tilt/3(fErrorReduction)
  Data Store Read23/1 -> pid2ControllerStep(oPidDataRpmCtrll_tilt/17(fKp)
  pid2ControllerStep(oPidDataRpmCtrll_tilt/3(fDTerm) -> Data Store Write2/1
  pid2ControllerStep(oPidDataRpmCtrll_tilt/2(fITerm) -> Data Store Write1/1
  Data Store Read19/1 -> pid2ControllerStep(oPidDataRpmCtrll_tilt/12(fIntegratorLeakFactor)
  pid2ControllerStep(oPidDataRpmCtrll_tilt/1(iLargeErrorPresent) -> Data Store Write/1
  Data Store Read7/1 -> pid2ControllerStep(oPidDataRpmCtrll_tilt/1(fActual)
  Constant1/1 -> pid2ControllerStep(oPidDataRpmCtrll_tilt/14(fActualDt)
  Data Store Read4/1 -> pid2ControllerStep(oPidDataRpmCtrll_tilt/20(fpState)
  Data Store Read16/1 -> pid2ControllerStep(oPidDataRpmCtrll_tilt/10(fIntMax)
  Data Store Read9/1 -> pid2ControllerStep(oPidDataRpmCtrll_tilt/4(fLargeErrorThresholdPositive)
  Data Store Read3/1 -> pid2ControllerStep(oPidDataRpmCtrll_tilt/18(fOutMax)
  pid2ControllerStep(oPidDataRpmCtrll_tilt/6(*fpState) -> Data Store Write5/1
  Data Store Read12/1 -> pid2ControllerStep(oPidDataRpmCtrll_tilt/6(fBlankingMaxError)
  Data Store Read24/1 -> pid2ControllerStep(oPidDataRpmCtrll_tilt/19(fOutMin)
  Data Store Read21/1 -> pid2ControllerStep(oPidDataRpmCtrll_tilt/15(fDMax)

== system Target_Control_System/Target_Control_System/MainLoop/tiltMotor_mainLoop/mainTask_tilt/motorTaskMainFastStep(&oTilt)/Control Loops - Tilt/Speed Controller Tilt/PIcontroller_sensorlessDrives ==
  oRampDataOmegaERef_.fRampOut : Inport
  Enable : EnablePort
  Constant2 : Constant  OutDataTypeStr=single  SampleTime=-1
  Data Store Read1 : DataStoreRead  DataStoreName=oTilt  DataStoreElements=oTilt.oMot_.oParam_.oPiDataRpm_.oParameter_.fKp_  IndexOptions=Index vector (dialog)  Indices=1  OutputSizes=1
  Data Store Read11 : DataStoreRead  DataStoreName=oTilt  DataStoreElements=oTilt.oMot_.oParam_.oPiDataRpm_.oParameter_.fLoopDt_  IndexOptions=Index vector (dialog)  Indices=1  OutputSizes=1
  Data Store Read13 : DataStoreRead  DataStoreName=oTilt  DataStoreElements=oTilt.oMot_.oParam_.oPiDataRpm_.oParameter_.fOutMin_  IndexOptions=Index vector (dialog)  Indices=1  OutputSizes=1
  Data Store Read2 : DataStoreRead  DataStoreName=oTilt  DataStoreElements=oTilt.oMot_.oParam_.oPiDataRpm_.oParameter_.fKi_  IndexOptions=Index vector (dialog)  Indices=1  OutputSizes=1
  Data Store Read25 : DataStoreRead  DataStoreName=oTilt  DataStoreElements=oTilt.oMot_.oParam_.oPiDataRpm_.oParameter_.fOutMax_  IndexOptions=Index vector (dialog)  Indices=1  OutputSizes=1
  Data Store Read26 : DataStoreRead  DataStoreName=oTilt  DataStoreElements=oTilt.oMot_.oParam_.oPiDataRpm_.fState_  IndexOptions=Index vector (dialog)  Indices=1  OutputSizes=1
  Data Store Read27 : DataStoreRead  DataStoreName=oTilt  DataStoreElements=oTilt.oMot_.oIn_.fOmegaEObserverLpf2_  IndexOptions=Index vector (dialog)  Indices=1  OutputSizes=1
  Data Store Read5 : DataStoreRead  DataStoreName=oTilt  DataStoreElements=oTilt.oMot_.oParam_.oPiDataRpm_.oParameter_.fIntMax_  IndexOptions=Index vector (dialog)  Indices=1  OutputSizes=1
  Data Store Read6 : DataStoreRead  DataStoreName=oTilt  DataStoreElements=oTilt.oMot_.oParam_.oPiDataRpm_.oParameter_.fIntMin_  IndexOptions=Index vector (dialog)  Indices=1  OutputSizes=1
  Data Store Write4 : DataStoreWrite  DataStoreName=oTilt  DataStoreElements=oTilt.oMot_.oState_.fIqRefFromSpeedController_  IndexOptions=Index vector (dialog)  Indices=1  OutputSizes=1
  Data Store Write5 : DataStoreWrite  DataStoreName=oTilt  DataStoreElements=oTilt.oMot_.oParam_.oPiDataRpm_.fState_  IndexOptions=Index vector (dialog)  Indices=1  OutputSizes=1
  PI Speed Controller : Subsystem
  fIqRefFromSpeedController : Outport
  wires:
  PI Speed Controller/2(*fpState) -> Data Store Write5/1
  PI Speed Controller/1(fOutput) -> Data Store Write4/1, fIqRefFromSpeedController/1
  oRampDataOmegaERef_.fRampOut/1 -> PI Speed Controller/1(fTarget)
  Data Store Read27/1 -> PI Speed Controller/2(fActual)
  Constant2/1 -> PI Speed Controller/5(fScale)
  Data Store Read26/1 -> PI Speed Controller/11(fState)
  Data Store Read13/1 -> PI Speed Controller/10(fOutMin)
  Data Store Read25/1 -> PI Speed Controller/8(fOutMax)
  Data Store Read6/1 -> PI Speed Controller/9(fIntMin)
  Data Store Read5/1 -> PI Speed Controller/7(fIntMax)
  Data Store Read11/1 -> PI Speed Controller/6(fLoopDt)
  Data Store Read2/1 -> PI Speed Controller/4(fKi)
  Data Store Read1/1 -> PI Speed Controller/3(fKp)

== system Target_Control_System/Target_Control_System/MainLoop/tiltMotor_mainLoop/mainTask_tilt/motorTaskMainFastStep(&oTilt)/Control Loops - Tilt/Speed Controller Tilt/Set Iq Ref Tilt ==
  fIqRefFromSpeedController : Inport
  Enable : EnablePort
  Data Store Read : DataStoreRead  DataStoreName=oTilt  DataStoreElements=oTilt.oMot_.oState_.oFilterDataForSpeedControlIqRef_.afConstantsA_.h0  IndexOptions=Index vector (dialog)  Indices=1  OutputSizes=1
  Data Store Read1 : DataStoreRead  DataStoreName=oTilt  DataStoreElements=oTilt.oMot_.oState_.oFilterDataForSpeedControlIqRef_.afConstantsA_.h1  IndexOptions=Index vector (dialog)  Indices=1  OutputSizes=1
  Data Store Read2 : DataStoreRead  DataStoreName=oTilt  DataStoreElements=oTilt.oMot_.oState_.oFilterDataForSpeedControlIqRef_.afConstantsA_.h2  IndexOptions=Index vector (dialog)  Indices=1  OutputSizes=1
  Data Store Read3 : DataStoreRead  DataStoreName=oTilt  DataStoreElements=oTilt.oMot_.oState_.oFilterDataForSpeedControlIqRef_.afConstantsB_.h0  IndexOptions=Index vector (dialog)  Indices=1  OutputSizes=1
  Data Store Read4 : DataStoreRead  DataStoreName=oTilt  DataStoreElements=oTilt.oMot_.oState_.oFilterDataForSpeedControlIqRef_.afConstantsB_.h1  IndexOptions=Index vector (dialog)  Indices=1  OutputSizes=1
  Data Store Read5 : DataStoreRead  DataStoreName=oTilt  DataStoreElements=oTilt.oMot_.oState_.oFilterDataForSpeedControlIqRef_.afConstantsB_.h2  IndexOptions=Index vector (dialog)  Indices=1  OutputSizes=1
  Data Store Read6 : DataStoreRead  DataStoreName=oTilt  DataStoreElements=oTilt.oMot_.oState_.oFilterDataForSpeedControlIqRef_.afPreviousInputs_.h0  IndexOptions=Index vector (dialog)  Indices=1  OutputSizes=1
  Data Store Read7 : DataStoreRead  DataStoreName=oTilt  DataStoreElements=oTilt.oMot_.oState_.oFilterDataForSpeedControlIqRef_.afPreviousInputs_.h1  IndexOptions=Index vector (dialog)  Indices=1  OutputSizes=1
  Data Store Read8 : DataStoreRead  DataStoreName=oTilt  DataStoreElements=oTilt.oMot_.oState_.oFilterDataForSpeedControlIqRef_.afPreviousOutputs_.h0  IndexOptions=Index vector (dialog)  Indices=1  OutputSizes=1
  Data Store Read9 : DataStoreRead  DataStoreName=oTilt  DataStoreElements=oTilt.oMot_.oState_.oFilterDataForSpeedControlIqRef_.afPreviousOutputs_.h1  IndexOptions=Index vector (dialog)  Indices=1  OutputSizes=1
  Data Store Write1 : DataStoreWrite  DataStoreName=oTilt  DataStoreElements=oTilt.oMot_.oState_.oFilterDataForSpeedControlIqRef_.fFilterOutput_  IndexOptions=Index vector (dialog)  Indices=1  OutputSizes=1
  Data Store Write2 : DataStoreWrite  DataStoreName=oTilt  DataStoreElements=oTilt.oMot_.oState_.oFilterDataForSpeedControlIqRef_.afPreviousOutputs_.h0  IndexOptions=Index vector (dialog)  Indices=1  OutputSizes=1
  Data Store Write3 : DataStoreWrite  DataStoreName=oTilt  DataStoreElements=oTilt.oMot_.oState_.oFilterDataForSpeedControlIqRef_.afPreviousOutputs_.h1  IndexOptions=Index vector (dialog)  Indices=1  OutputSizes=1
  Data Store Write4 : DataStoreWrite  DataStoreName=oTilt  DataStoreElements=oTilt.oMot_.oState_.oFilterDataForSpeedControlIqRef_.afPreviousInputs_.h0  IndexOptions=Index vector (dialog)  Indices=1  OutputSizes=1
  Data Store Write5 : DataStoreWrite  DataStoreName=oTilt  DataStoreElements=oTilt.oMot_.oState_.oFilterDataForSpeedControlIqRef_.afPreviousInputs_.h1  IndexOptions=Index vector (dialog)  Indices=1  OutputSizes=1
  Data Store Write6 : DataStoreWrite  DataStoreName=oTilt  DataStoreElements=oTilt.oMot_.oState_.fIqRefBeforeRamp_  IndexOptions=Index vector (dialog)  Indices=1  OutputSizes=1
  softwareIirFilterStep() : Subsystem
  wires:
  softwareIirFilterStep()/1(*afPreviousInputs1) -> Data Store Write5/1
  softwareIirFilterStep()/2(*afPreviousInputs0) -> Data Store Write4/1
  softwareIirFilterStep()/3(*afPreviousOutputs1) -> Data Store Write3/1
  softwareIirFilterStep()/4(*afPreviousOutputs0) -> Data Store Write2/1
  softwareIirFilterStep()/5(fFilterOutput) -> Data Store Write1/1
  Data Store Read6/1 -> softwareIirFilterStep()/8(afPreviousInputs0)
  Data Store Read7/1 -> softwareIirFilterStep()/9(afPreviousInputs1)
  Data Store Read8/1 -> softwareIirFilterStep()/10(afPreviousOutputs0)
  Data Store Read9/1 -> softwareIirFilterStep()/11(afPreviousOutputs1)
  Data Store Read2/1 -> softwareIirFilterStep()/7(afConstantsA2)
  Data Store Read1/1 -> softwareIirFilterStep()/6(afConstantsA1)
  Data Store Read/1 -> softwareIirFilterStep()/5(afConstantsA0)
  Data Store Read3/1 -> softwareIirFilterStep()/2(afConstantsB0)
  Data Store Read4/1 -> softwareIirFilterStep()/3(afConstantsB1)
  Data Store Read5/1 -> softwareIirFilterStep()/4(afConstantsB2)
  fIqRefFromSpeedController/1 -> softwareIirFilterStep()/1(newInput), Data Store Write6/1

== system Target_Control_System/Target_Control_System/MainLoop/tiltMotor_mainLoop/mainTask_tilt/motorTaskMainFastStep(&oTilt)/Mechanical System - Tilt/processSensors(&oPitch)/Auxiliary sensor ==
  note: // Only process this if the sensor is actually there (mostly to save time for the QI).
  Enable : EnablePort
  Add1 : Sum
  Add3 : Sum
  Constant1 : Constant  Value=pi  OutDataTypeStr=single  SampleTime=-1
  Constant2 : Constant  Value=2*pi  OutDataTypeStr=single  SampleTime=-1
  Constant4 : Constant  Value=pi  OutDataTypeStr=single  SampleTime=-1
  Constant5 : Constant  Value=2*pi  OutDataTypeStr=single  SampleTime=-1
  Data Store Read1 : DataStoreRead  DataStoreName=oTilt  DataStoreElements=oTilt.oMot_.oState_.oPosSensor_.iAuxiliarySensorInverseDirection_  IndexOptions=Index vector (dialog)  Indices=1  OutputSizes=1
  Data Store Read2 : DataStoreRead  DataStoreName=oTilt  DataStoreElements=oTilt.oMot_.oIn_.oAdcData_.fAuxiliaryEncoderFloat_  IndexOptions=Index vector (dialog)  Indices=1  OutputSizes=1
  Data Store Read3 : DataStoreRead  DataStoreName=oTilt  DataStoreElements=oTilt.oMot_.oState_.oPosSensor_.fActuatorSensorOffsetAngle_  IndexOptions=Index vector (dialog)  Indices=1  OutputSizes=1
  Data Store Write1 : DataStoreWrite  DataStoreName=oTilt  DataStoreElements=oTilt.oMot_.oState_.oPosSensor_.fAuxiliaryAngleFromSensor_  IndexOptions=Index vector (dialog)  Indices=1  OutputSizes=1
  Subtract1 : Sum  Inputs=+-
  Subtract2 : Sum  Inputs=+-
  Subtract6 : Sum  Inputs=-+
  Switch1 : Switch  Threshold=-pi/2.0
  Switch2 : Switch  Criteria=u2 > Threshold
  Switch3 : Switch  Criteria=u2 > Threshold  Threshold=1.5*pi
  wires:
  Switch3/1 -> Data Store Write1/1
  Data Store Read2/1 -> Subtract1/2, Subtract2/1
  Data Store Read3/1 -> Add1/1
  Constant5/1 -> Add3/2
  Subtract2/1 -> Switch2/3
  Data Store Read1/1 -> Switch2/2
  Add3/1 -> Switch1/3
  Add1/1 -> Subtract6/2, Add3/1, Switch1/2, Switch1/1, Switch3/2
  Subtract6/1 -> Switch3/1
  Switch2/1 -> Add1/2
  Switch1/1 -> Switch3/3
  Subtract1/1 -> Switch2/1
  Constant2/1 -> Subtract6/1
  Constant1/1 -> Subtract2/2
  Constant4/1 -> Subtract1/1

== system Target_Control_System/Target_Control_System/MainLoop/tiltMotor_mainLoop/mainTask_tilt/motorTaskMainFastStep(&oTilt)/Mechanical System - Tilt/processSensors(&oPitch)/Input (motor) side sensor ==
  note: // Ensure the angle is within -pi/2 to pi*1.5 (no loop needed, assuming 'fActuatorSensorOffsetAngle_' is within -pi to pi)
      |    // The reason for this 'skewed' wrap around angle: the tilt sensor on the linkage style tilts moves between 0 and 200 deg,
      |    // so it'd be mighty convenient if it doesn't wrap around at 180 deg. The flaps have a similar situation.
      |    // For pivot style tilt and VP, the sensor moves between -15 deg and 100 deg at most, so the the shifted wrapping point is a non-issue.
  note: // In the tilt motor on nacelles 1 and 4-6, the sensor read head is mounted to the gearbox output shaft.
      | // For every full motor rotation, the read head moves by 1/160*360 degrees = 2.25 degrees w.r.t the stator.
      | // (So with our 20 pole pairs, that is 45 degrees electrical.)
      | // We have to adjust the offset for this.
  note: //Note to future self: there is a slim chance that 'opStates->oPosSensor_.oGbx_.fCurrentOutputAngle_'
      | may need to be multiplied by -1.0F for certain hardware assemblies. Just keep it in mind.
  " " : Subsystem
  Add5 : Sum
  Add6 : Sum
  Compute Speed From Sensor : Subsystem
  Constant15 : Constant  Value=pi  OutDataTypeStr=single  SampleTime=-1
  Constant18 : Constant  Value=pi  OutDataTypeStr=single  SampleTime=-1
  Data Store Read1 : DataStoreRead  DataStoreName=oTilt  DataStoreElements=oTilt.oMot_.oState_.oPosSensor_.iMotorSensorInverseDirection_  IndexOptions=Index vector (dialog)  Indices=1  OutputSizes=1
  Data Store Read2 : DataStoreRead  DataStoreName=oTilt  DataStoreElements=oTilt.oMot_.oIn_.oAdcData_.fMotorEncoderFloat_  IndexOptions=Index vector (dialog)  Indices=1  OutputSizes=1
  Data Store Read3 : DataStoreRead  DataStoreName=oTilt  DataStoreElements=oTilt.oMot_.oState_.oPosSensor_.fAngleElecFromSensorOffset_  IndexOptions=Index vector (dialog)  Indices=1  OutputSizes=1
  Data Store Read4 : DataStoreRead  DataStoreName=oTilt  DataStoreElements=oTilt.oMot_.oParam_.fOneOverSensorPolepairs_  IndexOptions=Index vector (dialog)  Indices=1  OutputSizes=1
  Data Store Read5 : DataStoreRead  DataStoreName=oTilt  DataStoreElements=oTilt.oMot_.oState_.oPosSensor_.iAngleElecFromSensorNumOfIdenticalValues_  IndexOptions=Index vector (dialog)  Indices=1  OutputSizes=1
  Data Store Read6 : DataStoreRead  DataStoreName=oTilt  DataStoreElements=oTilt.oMot_.oState_.oPosSensor_.iTiltReadheadCompensationEnabled_  IndexOptions=Index vector (dialog)  Indices=1  OutputSizes=1
  Data Store Read7 : DataStoreRead  DataStoreName=oTilt  DataStoreElements=oTilt.oMot_.oParam_.fPolePairs_  IndexOptions=Index vector (dialog)  Indices=1  OutputSizes=1
  Data Store Write2 : DataStoreWrite  DataStoreName=oTilt  DataStoreElements=oTilt.oMot_.oState_.oPosSensor_.fAngleMechMotorFromSensor_  IndexOptions=Index vector (dialog)  Indices=1  OutputSizes=1
  Data Store Write3 : DataStoreWrite  DataStoreName=oTilt  DataStoreElements=oTilt.oMot_.oState_.oPosSensor_.iAngleMechToElecWrappings_  IndexOptions=Index vector (dialog)  Indices=1  OutputSizes=1
  Data Store Write39 : DataStoreWrite  DataStoreName=oTilt  DataStoreElements=oTilt.oMot_.oState_.oPosSensor_.fAngleElecFromSensor_  IndexOptions=Index vector (dialog)  Indices=1  OutputSizes=1
  Data Store Write4 : DataStoreWrite  DataStoreName=oTilt  DataStoreElements=oTilt.oMot_.oState_.oPosSensor_.fOmegaEFromSensor_  IndexOptions=Index vector (dialog)  Indices=1  OutputSizes=1
  Data Store Write41 : DataStoreWrite  DataStoreName=oTilt  DataStoreElements=oTilt.oMot_.oState_.oPosSensor_.fAngleElecFromSensorPrevious_  IndexOptions=Index vector (dialog)  Indices=1  OutputSizes=1
  PosSensorProcess_altImplementations : Subsystem  Commented=on
  Product : Product  Inputs=3
  Stuck Sensor Detection : Subsystem
  Subtract6 : Sum  Inputs=+-
  Subtract7 : Sum  Inputs=+-
  Switch14 : Switch  Criteria=u2 > Threshold
  Switch16 : Switch  Criteria=u2 > Threshold
  Unit Delay : UnitDelay  SampleTime=-1  HasFrameUpgradeWarning=on
  updateGbxOutput : Subsystem
  wires:
  Switch16/1 -> Product/1
  Data Store Read6/1 -> Switch16/2
  Data Store Read3/1 -> Add6/2
  Data Store Read1/1 -> Switch14/2
  Add6/1 -> " "/1(input_angle)  "angle_elec_unwrapped"
  Add5/1 -> Switch16/1
  Switch14/1 -> updateGbxOutput/1(fNewInputAngle), Switch16/3, Add5/2, Data Store Write2/1  "fAngleMechMotorFromSensor"
  " "/2(wrapped_angle) -> Unit Delay/1, Compute Speed From Sensor/2(fAngleElecFromSensor), Stuck Sensor Detection/1(fAngleElecFromSensor), Data Store Write39/1  "fAngleElecFromSensor"
  " "/1(rev_count) -> Data Store Write3/1
  Data Store Read2/1 -> Subtract7/1, Subtract6/2  "fMotorEncoderFloat"
  Product/1 -> Add6/1
  Data Store Read5/1 -> Stuck Sensor Detection/2(NumOfIdenticalValues)
  Data Store Read4/1 -> Product/3
  Compute Speed From Sensor/1(fOmegaEFromSensor) -> Data Store Write4/1
  Constant15/1 -> Subtract7/2
  Subtract6/1 -> Switch14/1
  Data Store Read7/1 -> Product/2
  Unit Delay/1 -> Stuck Sensor Detection/3(fAngleElecFromSensorPrevious), Compute Speed From Sensor/1(fAngleElecFromSensorPrevious)
  Compute Speed From Sensor/2(AngleCurrent) -> Data Store Write41/1
  Constant18/1 -> Subtract6/1
  updateGbxOutput/1(fCurrentOutputAngle) -> Add5/1
  Subtract7/1 -> Switch14/3
